simulink model "simexa25"  (Simulink 2.09)
settings: Solver=ode45  StartTime=0.0  StopTime=5.0  RelTol=1e-5  AbsTol=1e-6
settings Model: ConsistencyChecking=off  RTWTemplateMakefile=grt_vc.tmf

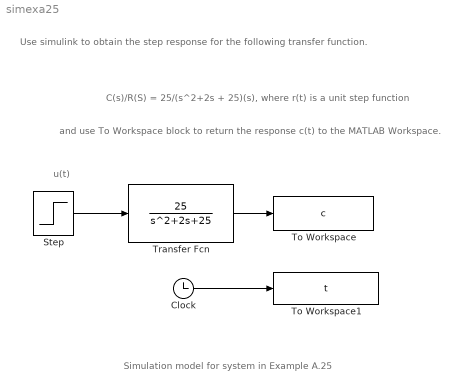
== system simexa25 ==
  note: Simulation model for system in Example A.25
  note: C(s)/R(S) = 25/(s^2+2s + 25)(s), where r(t) is a unit step function
  note: Use simulink to obtain the step response for the
      |    following transfer function.
  note: and use To Workspace block to return the response c(t) to the
      | MATLAB Workspace.
  note: u(t)
  Clock : Clock
  Step : Step  Time=1  Before=1  After=1
  To Workspace : ToWorkspace  VariableName=c  SampleTime=-1
  To Workspace1 : ToWorkspace  VariableName=t  SampleTime=-1
  Transfer Fcn : TransferFcn  Numerator=[25]  Denominator="[1  2   25]"
  wires:
  Clock/1 -> To Workspace1/1
  Step/1 -> Transfer Fcn/1
  Transfer Fcn/1 -> To Workspace/1
